simulink model "model_02_continuous"  (R2024b)
settings: Solver=VariableStepAuto  StartTime=0.0  StopTime=10.0  RelTol=1e-3
model workspace (MAT data in the model file):
  Km = 14.9
  Kp = 3
  Ts = 0.1
  tau = 0.174
settings Model: Creator=santi  LastModifiedBy=santi

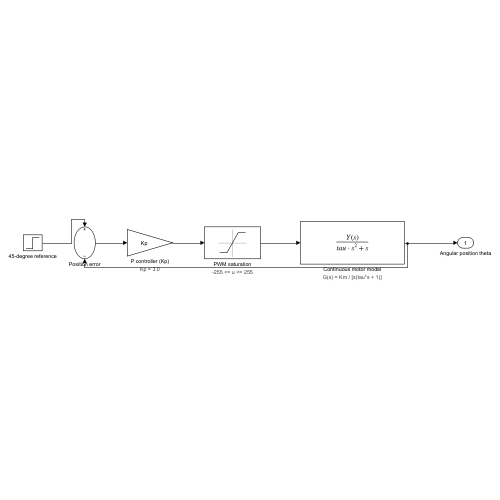
[thumbnail: Simulink's stored preview of the top-level diagram]
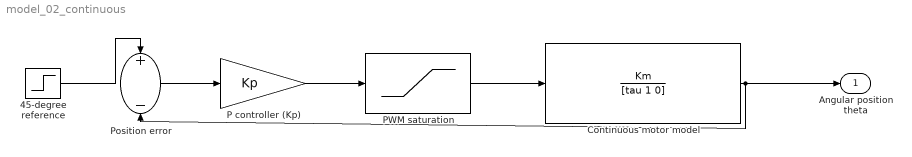
== system model_02_continuous ==
  45-degree reference : Step  After=45  SampleTime=0
  Continuous motor model : TransferFcn  Numerator=Km  Denominator=[tau 1 0]
      settings: AttributesFormatString=G(s) = Km / [s(tau*s + 1)]
  P controller (Kp) : Gain  Gain=Kp
      settings: AttributesFormatString=Kp = 3.0
  PWM saturation : Saturate  UpperLimit=255  LowerLimit=-255
      settings: AttributesFormatString=-255 <= u <= 255
  Position error : Sum  Inputs=+-
  Angular position theta : Outport
  wires:
  45-degree reference/1 -> Position error/1
  Position error/1 -> P controller (Kp)/1
  P controller (Kp)/1 -> PWM saturation/1
  PWM saturation/1 -> Continuous motor model/1
  Continuous motor model/1 -> Angular position theta/1, Position error/2
